simulink model "model"  (R2024b)
settings: Solver=ode4  StartTime=0.0  StopTime=simTime  FixedStep=sample_time  RelTol=1e-3
values from neighbouring files (symbols this model uses):
  gamma = 0.5    [init.m]
  k0 = 2    [init.m]
settings Model: Creator=kemal  LastModifiedBy=akdal

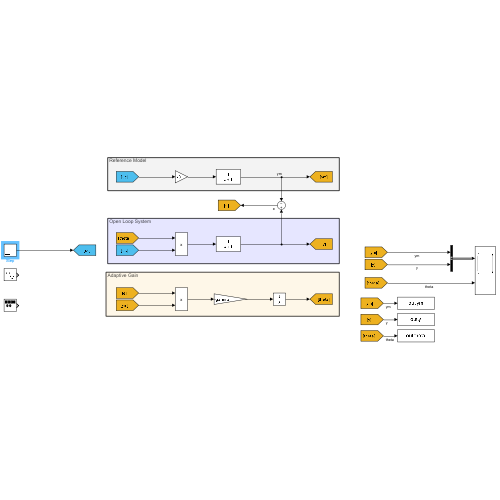
[thumbnail: Simulink's stored preview of the top-level diagram]
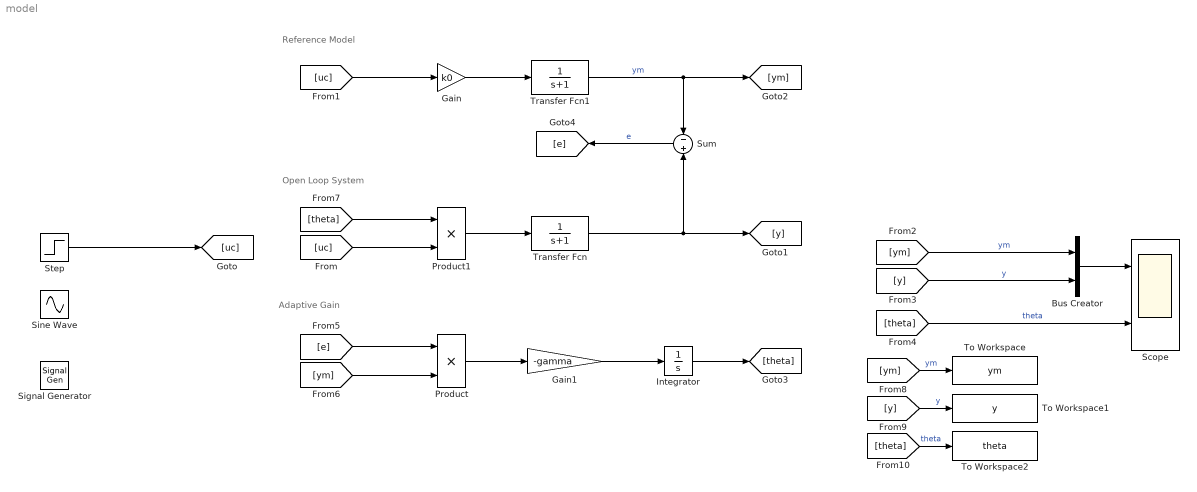
== system model ==
  note: Adaptive Gain
  note: Reference Model
  note: Open Loop System
  Bus Creator : BusCreator  Inputs=2
  Gain : Gain  Gain=k0
  Gain1 : Gain  Gain=-gamma
  Integrator : Integrator
  Product : Product
  Product1 : Product
  Scope : Scope  NumInputPorts=2
  Signal Generator : SignalGenerator  WaveForm=square  Units=rad/sec
  Sine Wave : Sin  Frequency=2*pi/5  SampleTime=0
  Step : Step  Time=0  SampleTime=0
  Sum : Sum  Inputs=-+
  To Workspace : ToWorkspace  VariableName=ym  SaveFormat=Timeseries  SampleTime=-1
  To Workspace1 : ToWorkspace  VariableName=y  SaveFormat=Timeseries  SampleTime=-1
  To Workspace2 : ToWorkspace  VariableName=theta  SaveFormat=Timeseries  SampleTime=-1
  Transfer Fcn : TransferFcn  Denominator=[1 1]
  Transfer Fcn1 : TransferFcn  Denominator=[1 1]
  wires:
  Gain/1 -> Transfer Fcn1/1
  Transfer Fcn1/1 -> Sum/1, [ym]  "ym"
  Transfer Fcn/1 -> [y], Sum/2
  Sum/1 -> [e]  "e"
  Product/1 -> Gain1/1
  Product1/1 -> Transfer Fcn/1
  Gain1/1 -> Integrator/1
  [uc] -> Product1/2
  Step/1 -> [uc]
  [uc] -> Gain/1
  [ym] -> Bus Creator/1  "ym"
  [y] -> Bus Creator/2  "y"
  Bus Creator/1 -> Scope/1
  [theta] -> Scope/2  "theta"
  Integrator/1 -> [theta]
  [e] -> Product/1
  [ym] -> Product/2
  [theta] -> Product1/1
  [ym] -> To Workspace/1  "ym"
  [y] -> To Workspace1/1  "y"
  [theta] -> To Workspace2/1  "theta"
